simulink model "jenkins_test"  (R2020b)
settings: Solver=VariableStepAuto  StartTime=0.0  StopTime=10.0  RelTol=1e-3
undefined symbols (not defined in the file): dv_Hyd_Pump_Green_Repress_InFlight_N3_Upper_Level, dv_Hyd_Pump_Green_Repress_OnGround_N3_Upper_Level, dv_Hyd_Pumps_Depress_NH_Hysteresis_Lower_Level
settings Model: Creator=IHADNQHN  LastModifiedBy=IHADNQHN

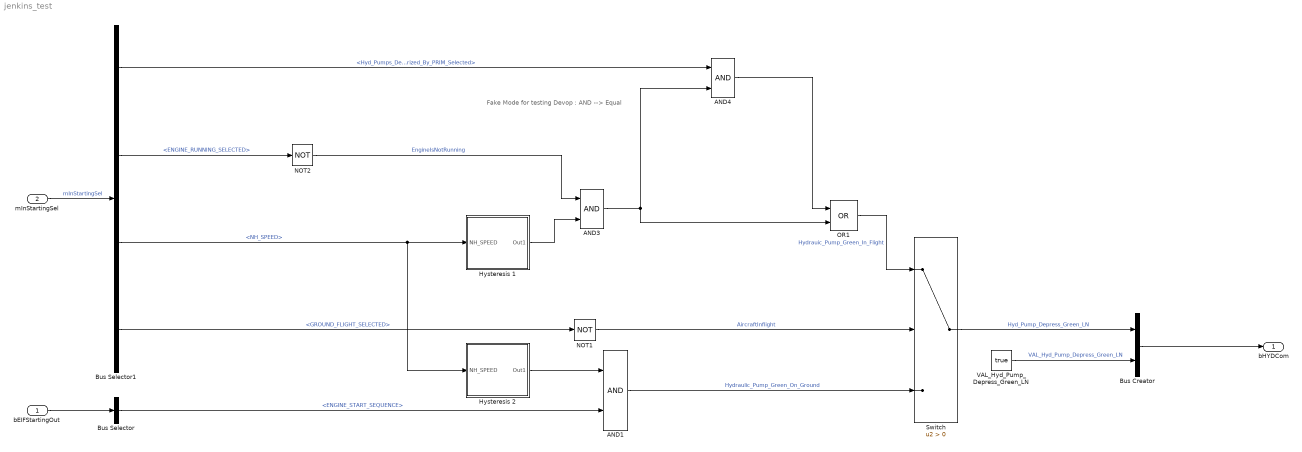
== system jenkins_test ==
  note: Fake Mode for testing Devop : AND --> Equal
  bEIFStartingOut : Inport
  mInStartingSel : Inport  Port=2
  AND1 : Logic  IconShape=distinctive  AllPortsSameDT=off  OutDataTypeStr=boolean
  AND3 : Logic  IconShape=distinctive  AllPortsSameDT=off  OutDataTypeStr=boolean
  AND4 : Logic  IconShape=distinctive  AllPortsSameDT=off  OutDataTypeStr=boolean
  Bus Creator : BusCreator  Inputs=2
  Bus Selector : BusSelector  OutputSignals=mStartSequence.ENGINE_START_SEQUENCE
  Bus Selector1 : BusSelector  OutputSignals=mPRIMSel.Hyd_Pumps_Depress_Authorized_By_PRIM_Selected,mEngineStatusSel.ENGINE_RUNNING_SELECTED,mEngineStatusSel.NH_SPEED,mGroundFlightStatusSel.GROUND_FLIGHT_SELECTED
  Hysteresis 1 : Subsystem
  Hysteresis 2 : Subsystem
  NOT1 : Logic  Operator=NOT  IconShape=distinctive  AllPortsSameDT=off  OutDataTypeStr=boolean
  NOT2 : Logic  Operator=NOT  IconShape=distinctive  AllPortsSameDT=off  OutDataTypeStr=boolean
  OR1 : Logic  Operator=OR  IconShape=distinctive  AllPortsSameDT=off  OutDataTypeStr=boolean
  Switch : Switch  Criteria=u2 > Threshold
  VAL_Hyd_Pump_Depress_Green_LN : Constant  Value=true
  bHYDCom : Outport
  wires:
  AND4/1 -> OR1/1
  OR1/1 -> Switch/1  "Hydrauic_Pump_Green_In_Flight"
  Switch/1 -> Bus Creator/1  "Hyd_Pump_Depress_Green_LN"
  Bus Selector/1 -> AND1/2  "<ENGINE_START_SEQUENCE>"
  Bus Selector1/1 -> AND4/1  "<Hyd_Pumps_Depress_Authorized_By_PRIM_Selected>"
  AND1/1 -> Switch/3  "Hydraulic_Pump_Green_On_Ground"
  Bus Selector1/3 -> Hysteresis 2/1(NH_SPEED), Hysteresis 1/1(NH_SPEED)  "<NH_SPEED>"
  bEIFStartingOut/1 -> Bus Selector/1
  NOT2/1 -> AND3/1  "EngineIsNotRunning"
  Bus Creator/1 -> bHYDCom/1
  Bus Selector1/2 -> NOT2/1  "<ENGINE_RUNNING_SELECTED>"
  Hysteresis 1/1(Out1) -> AND3/2
  AND3/1 -> OR1/2, AND4/2
  Hysteresis 2/1(Out1) -> AND1/1
  mInStartingSel/1 -> Bus Selector1/1  "mInStartingSel"
  Bus Selector1/4 -> NOT1/1  "<GROUND_FLIGHT_SELECTED>"
  VAL_Hyd_Pump_Depress_Green_LN/1 -> Bus Creator/2  "VAL_Hyd_Pump_Depress_Green_LN"
  NOT1/1 -> Switch/2  "AircraftInflight"

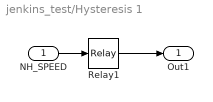
== system jenkins_test/Hysteresis 1 ==
  NH_SPEED : Inport
  Relay1 : Relay  OnSwitchValue=dv_Hyd_Pump_Green_Repress_InFlight_N3_Upper_Level  OffSwitchValue=dv_Hyd_Pumps_Depress_NH_Hysteresis_Lower_Level  OnOutputValue=0  OffOutputValue=1
  Out1 : Outport
  wires:
  Relay1/1 -> Out1/1
  NH_SPEED/1 -> Relay1/1

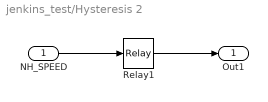
== system jenkins_test/Hysteresis 2 ==
  NH_SPEED : Inport
  Relay1 : Relay  OnSwitchValue=dv_Hyd_Pump_Green_Repress_OnGround_N3_Upper_Level  OffSwitchValue=dv_Hyd_Pumps_Depress_NH_Hysteresis_Lower_Level  OnOutputValue=0  OffOutputValue=1
  Out1 : Outport
  wires:
  Relay1/1 -> Out1/1
  NH_SPEED/1 -> Relay1/1
